simulink model "Model_with_controller"  (R2020a)
settings: Solver=VariableStepAuto  StartTime=0.0  StopTime=10.0  RelTol=1e-3
model workspace (MAT data in the model file):
  Ki = 1
  Kp = 1
values from neighbouring files (symbols this model uses):
  b = 50.0    [Data_dict.sldd]
  m = 1000.0    [Data_dict.sldd]
settings Model: Creator=Shivam  LastModifiedBy=Shivam

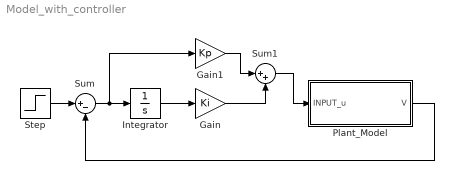
== system Model_with_controller ==
  Gain : Gain  Gain=Ki
  Gain1 : Gain  Gain=Kp
  Integrator : Integrator
  Plant_Model : Subsystem
  Step : Step  SampleTime=0
  Sum : Sum  Inputs=|+-
  Sum1 : Sum  Inputs=|++
  wires:
  Plant_Model/1(V) -> Sum/2
  Sum/1 -> Gain1/1, Integrator/1
  Integrator/1 -> Gain/1
  Gain1/1 -> Sum1/1
  Gain/1 -> Sum1/2
  Sum1/1 -> Plant_Model/1(INPUT_u)
  Step/1 -> Sum/1

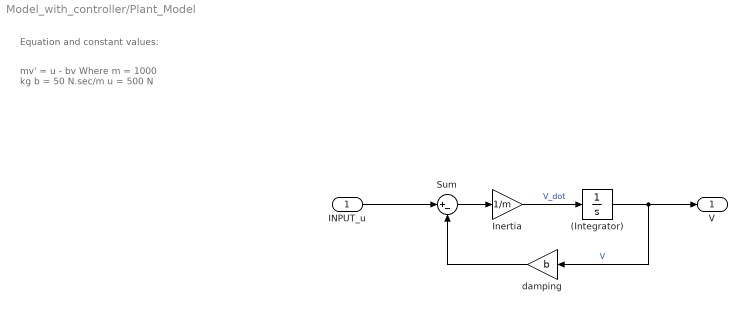
== system Model_with_controller/Plant_Model ==
  note: Equation and constant values:
  note: mv' = u - bv
      |
      | Where
      | m = 1000 kg
      | b = 50 N.sec/m
      | u = 500 N
  INPUT_u : Inport
  (Integrator) : Integrator
  Inertia : Gain  Gain=1/m
  Sum : Sum  Inputs=|+-
  damping : Gain  Gain=b
  V : Outport
  wires:
  INPUT_u/1 -> Sum/1
  (Integrator)/1 -> V/1, damping/1  "V"
  damping/1 -> Sum/2
  Inertia/1 -> (Integrator)/1  "V_dot"
  Sum/1 -> Inertia/1
